simulink library "SimulationLibrary"  (R2016b)
settings: Solver=ode45  StartTime=0.0  StopTime=10.0  RelTol=1e-3  EnableMultiTasking=on
values from neighbouring files (symbols this model uses):
  cassieEtherCatData = cassieEtherCat.getStructure    [simulationInitFcn.m]
  pelvisPosition = [0; 0; 1.01]    [simulationInitFcn.m]
undefined symbols (not defined in the file or in its folder): CassieParameters, leftFootDrive, leftLegMedulla, pelvisMedulla, X, Y, Z
libraries: sm_lib x86, SimulationLibrary x30, nesl_utility x18, Contact_Forces_Lib x2
(part 3 of 3)

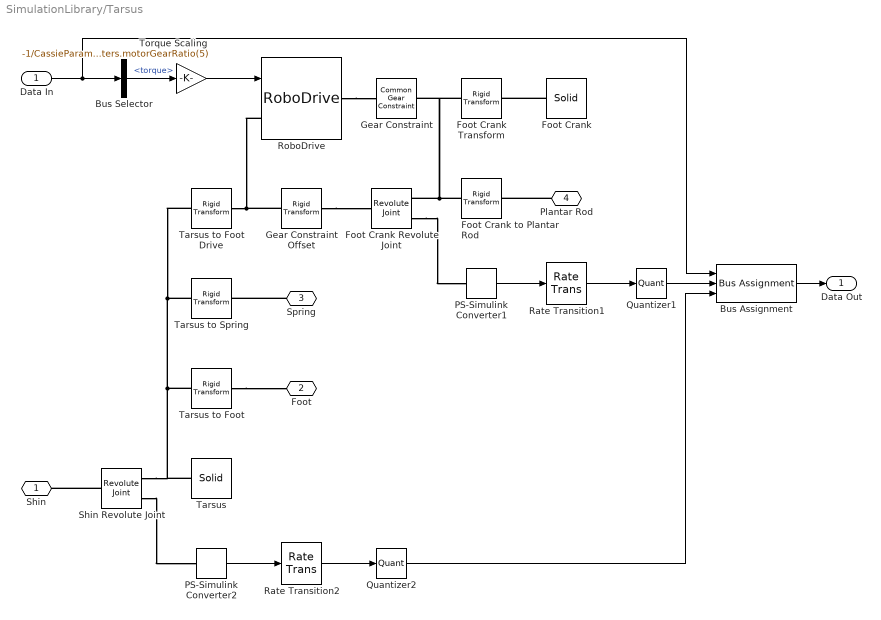
== system SimulationLibrary/Tarsus ==
  Data In : Inport  OutDataTypeStr=Bus: cassieEtherCatBus
  Bus Assignment : BusAssignment  AssignedSignals=leftFootDrive.inputs.position,leftLegMedulla.miscInputs.ankleJointEncoder
  Bus Selector : BusSelector  OutputSignals=leftFootDrive.outputs.torque
  Foot Crank : sm_lib/Body Elements/Solid  InertiaType=Custom  Mass=0.129  MassUnits=kg  CenterOfMass=[4.81; 0.02; -2.93]/1000  CenterOfMassUnits=m  MomentsOfInertia=[30.7; 57.05; 66.43]/1000000  MomentsOfInertiaUnits=kg*m^2  ProductsOfInertia=[0.0066; 2.62; 0.0019]/1000000  ProductsOfInertiaUnits=kg*m^2  DensityBased=on  Density=1000  DensityUnits=kg/(m^3)  DoExposeReferenceFrame=on  SerializedFrames=<Frames/>  GraphicType=FromGeometry  MarkerShape=Sphere  MarkerSize=10  GraphicVisPropType=AdvancedVisualProperties  GraphicDiffuseColor=simulationParameters.diffuseColor  GraphicSpecularColor=simulationParameters.specularColor  GraphicAmbientColor=simulationParameters.ambientColor  GraphicEmissiveColor=simulationParameters.emissiveColor  GraphicShininess=simulationParameters.shininess  GraphicOpacity=1  GeometryShape=FromFile  RectangleSize=[1 1]  RectangleSizeUnits=m  BrickDimensions=[1 1 1]  BrickDimensionUnits=m  CylinderRadius=1  CylinderRadiusUnits=m  CylinderLength=1  CylinderLengthUnits=m  SphereRadius=1  SphereRadiusUnits=m  EllipsoidRadii=[1 1 1]  EllipsoidRadiiUnits=m  ExtrusionCrossSection=[1 1; -1 1; -1 -1; 1 -1]  ExtrusionCrossSectionUnits=m  ExtrusionLength=1  ExtrusionLengthUnits=m  PolygonNumSides=3  PolygonOuterRadius=1  PolygonOuterRadiusUnits=m  ExtGeomFileType=STL  ExtGeomFileName=foot_crank.stl  ExtGeomFileUnits=m  RevolutionCrossSection=[1 1; 1 -1; 2 -1; 2 1]  RevolutionCrossSectionUnits=m  RevolutionExtent=Full  RevolutionAngle=180  RevolutionAngleUnits=deg
  Foot Crank Revolute Joint : sm_lib/Joints/Revolute Joint  SenseConstraintForce=off  SenseConstraintForceX=off  SenseConstraintForceY=off  SenseConstraintForceZ=off  SenseConstraintTorque=off  SenseConstraintTorqueX=off  SenseConstraintTorqueY=off  SenseConstraintTorqueZ=off  SenseTotalForce=off  SenseTotalForceX=off  SenseTotalForceY=off  SenseTotalForceZ=off  SenseTotalTorque=off  SenseTotalTorqueX=off  SenseTotalTorqueY=off  SenseTotalTorqueZ=off  CompositeWrenchDir=FollowerOnBase  CompositeWrenchFrame=BaseFrame  EquilibriumPosition=0  EquilibriumPositionUnits=deg  SpringStiffness=0  SpringStiffnessUnits=N*m/deg  DampingCoefficient=CassieParameters.motorViscousFrictionCoefficient(5)  DampingCoefficientUnits=N*m/(rad/s)  TorqueActuationMode=NoTorque  MotionActuationMode=ComputedMotion  SensePosition=on  SenseVelocity=off  SenseAcceleration=off  SenseTorqueForce=off  PositionTargetSpecify=on  PositionTargetPriority=High  PositionTargetValue=cassieEtherCatData.leftFootDrive.inputs.position  PositionTargetValueUnits=rad  VelocityTargetSpecify=on  VelocityTargetPriority=High  VelocityTargetValue=0  VelocityTargetValueUnits=rad/s
  Foot Crank Transform : sm_lib/Frames and Transforms/Rigid Transform  TranslationMethod=None  TranslationStandardOffset=0  TranslationLengthUnit=m  TranslationStandardAxis=+Z  TranslationCartesianOffset=[0 0 0]  TranslationROffset=0  TranslationROffsetUnits=m  TranslationZOffset=0  TranslationZOffsetUnits=m  TranslationThetaOffset=0  TranslationThetaOffsetUnits=deg  RotationMethod=StandardAxis  RotationAngleUnits=rad  RotationStandardAxis=+X  RotationAngle=0  RotationArbitraryAxis=[0 0 1]  FollAlignAxisA=+X  BaseAlignAxisA=+Y  FollAlignAxisB=+Y  BaseAlignAxisB=+Z  RotationSequenceAxes=FollowerAxes  RotationSequence=XYZ  RotationSequenceAngles=[90 0 0]  RotationSequenceAnglesUnits=deg  RotationMatrix=[1 0 0; 0 1 0; 0 0 1]
  Foot Crank to Plantar Rod : sm_lib/Frames and Transforms/Rigid Transform  TranslationMethod=Cartesian  TranslationStandardOffset=0  TranslationLengthUnit=m  TranslationStandardAxis=+Z  TranslationCartesianOffset=[55 0 -7.91]/1000  TranslationROffset=0  TranslationROffsetUnits=m  TranslationZOffset=0  TranslationZOffsetUnits=m  TranslationThetaOffset=0  TranslationThetaOffsetUnits=deg  RotationMethod=None  RotationAngleUnits=deg  RotationStandardAxis=+Z  RotationAngle=0.0  RotationArbitraryAxis=[0 0 1]  FollAlignAxisA=+X  BaseAlignAxisA=+Y  FollAlignAxisB=+Y  BaseAlignAxisB=+Z  RotationSequenceAxes=FollowerAxes  RotationSequence=XYZ  RotationSequenceAngles=[90 0 0]  RotationSequenceAnglesUnits=deg  RotationMatrix=[1 0 0; 0 1 0; 0 0 1]
  Gear Constraint : sm_lib/Gears and Couplings/Gears/Common Gear Constraint  GearType=External  SpecificationType=CenterDistanceRatio  CenterDistance=1e-6  CenterDistanceUnits=m  GearRatio=CassieParameters.motorGearRatio(5)  BaseGearRadius=10.0  BaseGearRadiusUnits=cm  FollGearRadius=10.0  FollGearRadiusUnits=cm  AssemblyGearRotation=Free
  Gear Constraint Offset : sm_lib/Frames and Transforms/Rigid Transform  TranslationMethod=StandardAxis  TranslationStandardOffset=1e-6  TranslationLengthUnit=m  TranslationStandardAxis=+Y  TranslationCartesianOffset=[0 0 0]  TranslationROffset=0  TranslationROffsetUnits=m  TranslationZOffset=0  TranslationZOffsetUnits=m  TranslationThetaOffset=0  TranslationThetaOffsetUnits=deg  RotationMethod=None  RotationAngleUnits=deg  RotationStandardAxis=+Z  RotationAngle=0.0  RotationArbitraryAxis=[0 0 1]  FollAlignAxisA=+X  BaseAlignAxisA=+Y  FollAlignAxisB=+Y  BaseAlignAxisB=+Z  RotationSequenceAxes=FollowerAxes  RotationSequence=XYX  RotationSequenceAngles=[0 0 0]  RotationSequenceAnglesUnits=deg  RotationMatrix=[1 0 0; 0 1 0; 0 0 1]
  PS-Simulink Converter1 : nesl_utility/PS-Simulink Converter  PhysicalDomain=network_engine_domain  SubClassName=ps_output  LeftPortType=input  RightPortType=output  PseudoPeriodic=off  Frequencies=[]  Unit=rad  AffineConversion=off
  PS-Simulink Converter2 : nesl_utility/PS-Simulink Converter  PhysicalDomain=network_engine_domain  SubClassName=ps_output  LeftPortType=input  RightPortType=output  PseudoPeriodic=off  Frequencies=[]  Unit=rad  AffineConversion=off
  Quantizer1 : Quantizer  QuantizationInterval=(2*pi)/(CassieParameters.motorEncoderTicks(5)*CassieParameters.motorGearRatio(5))
  Quantizer2 : Quantizer  QuantizationInterval=(2*pi)/CassieParameters.jointEncoderTicks(2)
  Rate Transition1 : RateTransition  Deterministic=off  OutPortSampleTime=CassieParameters.etherCatSampleTime
  Rate Transition2 : RateTransition  Deterministic=off  OutPortSampleTime=CassieParameters.etherCatSampleTime
  RoboDrive : SimulationLibrary/RoboDrive  model=50x8
  Shin Revolute Joint : sm_lib/Joints/Revolute Joint  SenseConstraintForce=off  SenseConstraintForceX=off  SenseConstraintForceY=off  SenseConstraintForceZ=off  SenseConstraintTorque=off  SenseConstraintTorqueX=off  SenseConstraintTorqueY=off  SenseConstraintTorqueZ=off  SenseTotalForce=off  SenseTotalForceX=off  SenseTotalForceY=off  SenseTotalForceZ=off  SenseTotalTorque=off  SenseTotalTorqueX=off  SenseTotalTorqueY=off  SenseTotalTorqueZ=off  CompositeWrenchDir=FollowerOnBase  CompositeWrenchFrame=BaseFrame  EquilibriumPosition=0  EquilibriumPositionUnits=deg  SpringStiffness=0  SpringStiffnessUnits=N*m/deg  DampingCoefficient=0  DampingCoefficientUnits=N*m/(deg/s)  TorqueActuationMode=NoTorque  MotionActuationMode=ComputedMotion  SensePosition=on  SenseVelocity=off  SenseAcceleration=off  SenseTorqueForce=off  PositionTargetSpecify=on  PositionTargetPriority=Low  PositionTargetValue=pi/2  PositionTargetValueUnits=rad  VelocityTargetSpecify=on  VelocityTargetPriority=High  VelocityTargetValue=0  VelocityTargetValueUnits=rad/s
  Tarsus : sm_lib/Body Elements/Solid  InertiaType=Custom  Mass=0.782  MassUnits=kg  CenterOfMass=[110.46; -30.58; -1.31]/1000  CenterOfMassUnits=m  MomentsOfInertia=[1125; 23138; 23947]/1000000  MomentsOfInertiaUnits=kg*m^2  ProductsOfInertia=[36.15; -63.29; -2878]/1000000  ProductsOfInertiaUnits=kg*m^2  DensityBased=on  Density=1000  DensityUnits=kg/(m^3)  DoExposeReferenceFrame=on  SerializedFrames=<Frames/>  GraphicType=FromGeometry  MarkerShape=Sphere  MarkerSize=10  GraphicVisPropType=AdvancedVisualProperties  GraphicDiffuseColor=simulationParameters.diffuseColor  GraphicSpecularColor=simulationParameters.specularColor  GraphicAmbientColor=simulationParameters.ambientColor  GraphicEmissiveColor=simulationParameters.emissiveColor  GraphicShininess=simulationParameters.shininess  GraphicOpacity=1.0  GeometryShape=FromFile  RectangleSize=[1 1]  RectangleSizeUnits=m  BrickDimensions=[1 1 1]  BrickDimensionUnits=m  CylinderRadius=1  CylinderRadiusUnits=m  CylinderLength=1  CylinderLengthUnits=m  SphereRadius=1  SphereRadiusUnits=m  EllipsoidRadii=[1 1 1]  EllipsoidRadiiUnits=m  ExtrusionCrossSection=[1 1; -1 1; -1 -1; 1 -1]  ExtrusionCrossSectionUnits=m  ExtrusionLength=1  ExtrusionLengthUnits=m  PolygonNumSides=3  PolygonOuterRadius=1  PolygonOuterRadiusUnits=m  ExtGeomFileType=STL  ExtGeomFileName=left_tarsus.stl  ExtGeomFileUnits=m  RevolutionCrossSection=[1 1; 1 -1; 2 -1; 2 1]  RevolutionCrossSectionUnits=m  RevolutionExtent=Full  RevolutionAngle=180  RevolutionAngleUnits=deg
  Tarsus to Foot : sm_lib/Frames and Transforms/Rigid Transform  TranslationMethod=Cartesian  TranslationStandardOffset=0  TranslationLengthUnit=m  TranslationStandardAxis=+Z  TranslationCartesianOffset=[408 -40 0]/1000  TranslationROffset=0  TranslationROffsetUnits=m  TranslationZOffset=0  TranslationZOffsetUnits=m  TranslationThetaOffset=0  TranslationThetaOffsetUnits=deg  RotationMethod=None  RotationAngleUnits=deg  RotationStandardAxis=+Z  RotationAngle=0.0  RotationArbitraryAxis=[0 0 1]  FollAlignAxisA=+X  BaseAlignAxisA=+Y  FollAlignAxisB=+Y  BaseAlignAxisB=+Z  RotationSequenceAxes=FollowerAxes  RotationSequence=XYZ  RotationSequenceAngles=[-90 0 0]  RotationSequenceAnglesUnits=deg  RotationMatrix=[1 0 0; 0 1 0; 0 0 1]
  Tarsus to Foot Drive : sm_lib/Frames and Transforms/Rigid Transform  TranslationMethod=Cartesian  TranslationStandardOffset=0  TranslationLengthUnit=m  TranslationStandardAxis=+Z  TranslationCartesianOffset=[58 -34 22.75]/1000  TranslationROffset=0  TranslationROffsetUnits=m  TranslationZOffset=0  TranslationZOffsetUnits=m  TranslationThetaOffset=0  TranslationThetaOffsetUnits=deg  RotationMethod=None  RotationAngleUnits=deg  RotationStandardAxis=+Z  RotationAngle=0  RotationArbitraryAxis=[0 0 1]  FollAlignAxisA=+X  BaseAlignAxisA=+Y  FollAlignAxisB=+Y  BaseAlignAxisB=+Z  RotationSequenceAxes=FollowerAxes  RotationSequence=XYZ  RotationSequenceAngles=[-90 0 0]  RotationSequenceAnglesUnits=deg  RotationMatrix=[1 0 0; 0 1 0; 0 0 1]
  Tarsus to Spring : sm_lib/Frames and Transforms/Rigid Transform  TranslationMethod=Cartesian  TranslationStandardOffset=0  TranslationLengthUnit=m  TranslationStandardAxis=+Z  TranslationCartesianOffset=[-12.69 -30.59 0.92]/1000  TranslationROffset=0  TranslationROffsetUnits=m  TranslationZOffset=0  TranslationZOffsetUnits=m  TranslationThetaOffset=0  TranslationThetaOffsetUnits=deg  RotationMethod=RotationSequence  RotationAngleUnits=deg  RotationStandardAxis=+Z  RotationAngle=0.0  RotationArbitraryAxis=[0 0 1]  FollAlignAxisA=+X  BaseAlignAxisA=+Y  FollAlignAxisB=+Y  BaseAlignAxisB=+Z  RotationSequenceAxes=BaseAxes  RotationSequence=ZYX  RotationSequenceAngles=[155.8, 0.315, 4.47]  RotationSequenceAnglesUnits=deg  RotationMatrix=eye(3)
  Torque Scaling : Gain  Gain=-1/CassieParameters.motorGearRatio(5)
  Shin : PMIOPort  Port=1  Side=Left
  Foot : PMIOPort  Port=2  Side=Right
  Spring : PMIOPort  Port=3  Side=Left
  Plantar Rod : PMIOPort  Port=4  Side=Right
  Data Out : Outport
  wires:
  Bus Assignment/1 -> Data Out/1
  Data In/1 -> Bus Selector/1, Bus Assignment/1
  PS-Simulink Converter2/1 -> Rate Transition2/1
  PS-Simulink Converter1/1 -> Rate Transition1/1
  Bus Selector/1 -> Torque Scaling/1  "<torque>"
  Torque Scaling/1 -> RoboDrive/1
  Rate Transition1/1 -> Quantizer1/1
  Quantizer1/1 -> Bus Assignment/2
  Rate Transition2/1 -> Quantizer2/1
  Quantizer2/1 -> Bus Assignment/3
  connections:
  Tarsus to Foot/RConn1 -- Foot/RConn1
  Spring/RConn1 -- Tarsus to Spring/RConn1
  Shin Revolute Joint/LConn1 -- Shin/RConn1
  Shin Revolute Joint/RConn2 -- PS-Simulink Converter2/LConn1
  Tarsus to Foot/LConn1 -- Shin Revolute Joint/RConn1 -- Tarsus/RConn1 -- Tarsus to Foot Drive/LConn1 -- Tarsus to Spring/LConn1
  Tarsus to Foot Drive/RConn1 -- Gear Constraint Offset/LConn1 -- RoboDrive/LConn1
  RoboDrive/RConn1 -- Gear Constraint/LConn1
  Gear Constraint Offset/RConn1 -- Foot Crank Revolute Joint/LConn1
  Foot Crank to Plantar Rod/LConn1 -- Foot Crank Revolute Joint/RConn1 -- Foot Crank Transform/LConn1 -- Gear Constraint/RConn1
  Plantar Rod/RConn1 -- Foot Crank to Plantar Rod/RConn1
  Foot Crank Revolute Joint/RConn2 -- PS-Simulink Converter1/LConn1
  Foot Crank/RConn1 -- Foot Crank Transform/RConn1

== system SimulationLibrary/Thigh ==
  Data In : Inport
  Thigh : sm_lib/Body Elements/Solid  InertiaType=Custom  Mass=5.52  MassUnits=kg  CenterOfMass=[59.46; 0.05; -35.81]/1000  CenterOfMassUnits=m  MomentsOfInertia=[17969; 56284; 49756]/1000000  MomentsOfInertiaUnits=kg*m^2  ProductsOfInertia=[-19.26; -11685; 283.6]/1000000  ProductsOfInertiaUnits=kg*m^2  DensityBased=on  Density=1000  DensityUnits=kg/(m^3)  DoExposeReferenceFrame=on  SerializedFrames=<Frames/>  GraphicType=FromGeometry  MarkerShape=Sphere  MarkerSize=10  MarkerSizeUnits=m  GraphicVisPropType=AdvancedVisualProperties  GraphicDiffuseColor=simulationParameters.diffuseColor  GraphicSpecularColor=simulationParameters.specularColor  GraphicAmbientColor=simulationParameters.ambientColor  GraphicEmissiveColor=simulationParameters.emissiveColor  GraphicShininess=simulationParameters.shininess  GraphicOpacity=1  GeometryShape=FromFile  RectangleSize=[1 1]  RectangleSizeUnits=m  BrickDimensions=[0.15 0.15 0.2]  BrickDimensionUnits=m  CylinderRadius=0.05  CylinderRadiusUnits=m  CylinderLength=0.1  CylinderLengthUnits=m  SphereRadius=1  SphereRadiusUnits=m  EllipsoidRadii=[1 1 1]  EllipsoidRadiiUnits=m  ExtrusionCrossSection=[1 1; -1 1; -1 -1; 1 -1]  ExtrusionCrossSectionUnits=m  ExtrusionLength=1  ExtrusionLengthUnits=m  PolygonNumSides=3  PolygonOuterRadius=1  PolygonOuterRadiusUnits=m  ExtGeomFileType=STL  ExtGeomFileName=left_thigh.stl  ExtGeomFileUnits=m  RevolutionCrossSection=[1 1; 1 -1; 2 -1; 2 1]  RevolutionCrossSectionUnits=m  RevolutionExtent=Full  RevolutionAngle=180  RevolutionAngleUnits=deg
  Thigh to Achilles : sm_lib/Frames and Transforms/Rigid Transform  TranslationMethod=Cartesian  TranslationStandardOffset=0  TranslationLengthUnit=m  TranslationStandardAxis=+Z  TranslationCartesianOffset=[0, 0, 0.045]  TranslationROffset=0  TranslationROffsetUnits=m  TranslationZOffset=0  TranslationZOffsetUnits=m  TranslationThetaOffset=0  TranslationThetaOffsetUnits=deg  RotationMethod=None  RotationAngleUnits=deg  RotationStandardAxis=+Z  RotationAngle=0.0  RotationArbitraryAxis=[0 0 1]  FollAlignAxisA=+X  BaseAlignAxisA=+Y  FollAlignAxisB=+Y  BaseAlignAxisB=+Z  RotationSequenceAxes=FollowerAxes  RotationSequence=XYX  RotationSequenceAngles=[0 0 0]  RotationSequenceAnglesUnits=deg  RotationMatrix=[1 0 0; 0 1 0; 0 0 1]
  Thigh to Knee : sm_lib/Frames and Transforms/Rigid Transform  TranslationMethod=Cartesian  TranslationStandardOffset=0  TranslationLengthUnit=m  TranslationStandardAxis=+Z  TranslationCartesianOffset=[0.12, 0, 0.0045]  TranslationROffset=0  TranslationROffsetUnits=m  TranslationZOffset=0  TranslationZOffsetUnits=m  TranslationThetaOffset=0  TranslationThetaOffsetUnits=deg  RotationMethod=None  RotationAngleUnits=deg  RotationStandardAxis=+Z  RotationAngle=0.0  RotationArbitraryAxis=[0 0 1]  FollAlignAxisA=+X  BaseAlignAxisA=+Y  FollAlignAxisB=+Y  BaseAlignAxisB=+Z  RotationSequenceAxes=FollowerAxes  RotationSequence=XYX  RotationSequenceAngles=[0 0 0]  RotationSequenceAnglesUnits=deg  RotationMatrix=[1 0 0; 0 1 0; 0 0 1]
  Hip : PMIOPort  Port=1  Side=Left
  Knee : PMIOPort  Port=2  Side=Right
  Achilles : PMIOPort  Port=3  Side=Right
  Data Out : Outport
  wires:
  Data In/1 -> Data Out/1
  connections:
  Hip/RConn1 -- Thigh to Knee/LConn1 -- Thigh to Achilles/LConn1 -- Thigh/RConn1
  Thigh to Knee/RConn1 -- Knee/RConn1
  Achilles/RConn1 -- Thigh to Achilles/RConn1

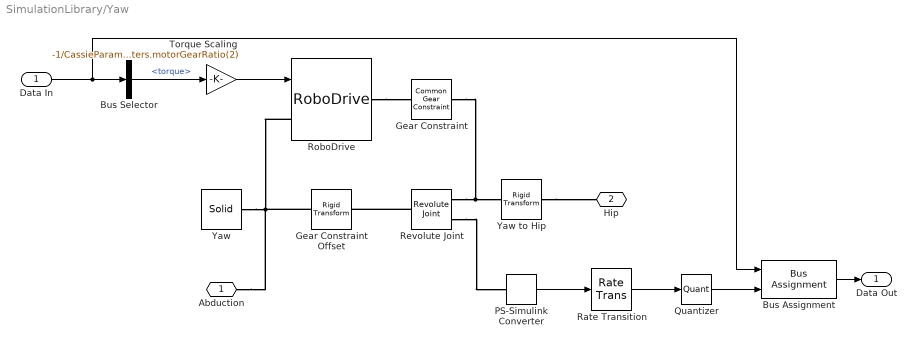
== system SimulationLibrary/Yaw ==
  Data In : Inport  OutDataTypeStr=Bus: cassieEtherCatBus
  Bus Assignment : BusAssignment  AssignedSignals=leftYawDrive.inputs.position
  Bus Selector : BusSelector  OutputSignals=leftYawDrive.outputs.torque
  Gear Constraint : sm_lib/Gears and Couplings/Gears/Common Gear Constraint  GearType=External  SpecificationType=CenterDistanceRatio  CenterDistance=1e-6  CenterDistanceUnits=m  GearRatio=CassieParameters.motorGearRatio(2)  BaseGearRadius=10.0  BaseGearRadiusUnits=cm  FollGearRadius=10.0  FollGearRadiusUnits=cm  AssemblyGearRotation=Free
  Gear Constraint Offset : sm_lib/Frames and Transforms/Rigid Transform  TranslationMethod=StandardAxis  TranslationStandardOffset=1e-6  TranslationLengthUnit=m  TranslationStandardAxis=+Y  TranslationCartesianOffset=[0 0 0]  TranslationROffset=0  TranslationROffsetUnits=m  TranslationZOffset=0  TranslationZOffsetUnits=m  TranslationThetaOffset=0  TranslationThetaOffsetUnits=deg  RotationMethod=None  RotationAngleUnits=deg  RotationStandardAxis=+Z  RotationAngle=0.0  RotationArbitraryAxis=[0 0 1]  FollAlignAxisA=+X  BaseAlignAxisA=+Y  FollAlignAxisB=+Y  BaseAlignAxisB=+Z  RotationSequenceAxes=FollowerAxes  RotationSequence=XYX  RotationSequenceAngles=[0 0 0]  RotationSequenceAnglesUnits=deg  RotationMatrix=[1 0 0; 0 1 0; 0 0 1]
  PS-Simulink Converter : nesl_utility/PS-Simulink Converter  PhysicalDomain=network_engine_domain  SubClassName=ps_output  LeftPortType=input  RightPortType=output  PseudoPeriodic=off  Frequencies=[]  Unit=rad  AffineConversion=off
  Quantizer : Quantizer  QuantizationInterval=(2*pi)/(CassieParameters.motorEncoderTicks(2)*CassieParameters.motorGearRatio(2))
  Rate Transition : RateTransition  Deterministic=off  OutPortSampleTime=CassieParameters.etherCatSampleTime
  Revolute Joint : sm_lib/Joints/Revolute Joint  SenseConstraintForce=off  SenseConstraintForceX=off  SenseConstraintForceY=off  SenseConstraintForceZ=off  SenseConstraintTorque=off  SenseConstraintTorqueX=off  SenseConstraintTorqueY=off  SenseConstraintTorqueZ=off  SenseTotalForce=off  SenseTotalForceX=off  SenseTotalForceY=off  SenseTotalForceZ=off  SenseTotalTorque=off  SenseTotalTorqueX=off  SenseTotalTorqueY=off  SenseTotalTorqueZ=off  CompositeWrenchDir=FollowerOnBase  CompositeWrenchFrame=BaseFrame  EquilibriumPosition=0  EquilibriumPositionUnits=rad  SpringStiffness=0  SpringStiffnessUnits=N*m/rad  DampingCoefficient=CassieParameters.motorViscousFrictionCoefficient(2)  DampingCoefficientUnits=N*m/(rad/s)  TorqueActuationMode=NoTorque  MotionActuationMode=ComputedMotion  SensePosition=on  SenseVelocity=off  SenseAcceleration=off  SenseTorqueForce=off  PositionTargetSpecify=on  PositionTargetPriority=High  PositionTargetValue=cassieEtherCatData.leftYawDrive.inputs.position  PositionTargetValueUnits=rad  VelocityTargetSpecify=on  VelocityTargetPriority=High  VelocityTargetValue=0  VelocityTargetValueUnits=rad/s
  RoboDrive : SimulationLibrary/RoboDrive  model=85x13
  Torque Scaling : Gain  Gain=-1/CassieParameters.motorGearRatio(2)
  Yaw : sm_lib/Body Elements/Solid  InertiaType=Custom  Mass=1.82  MassUnits=kg  CenterOfMass=[25.7; 0.1; 17.93]/1000  CenterOfMassUnits=m  MomentsOfInertia=[2722; 5586; 4638]/1000000  MomentsOfInertiaUnits=kg*m^2  ProductsOfInertia=[2.61; 1.53; 0.703]/1000000  ProductsOfInertiaUnits=kg*m^2  DensityBased=on  Density=1000  DensityUnits=kg/(m^3)  DoExposeReferenceFrame=on  SerializedFrames=<Frames/>  GraphicType=FromGeometry  MarkerShape=Sphere  MarkerSize=10  MarkerSizeUnits=m  GraphicVisPropType=AdvancedVisualProperties  GraphicDiffuseColor=simulationParameters.diffuseColor  GraphicSpecularColor=simulationParameters.specularColor  GraphicAmbientColor=simulationParameters.ambientColor  GraphicEmissiveColor=simulationParameters.emissiveColor  GraphicShininess=simulationParameters.shininess  GraphicOpacity=1  GeometryShape=FromFile  RectangleSize=[1 1]  RectangleSizeUnits=m  BrickDimensions=[0.15 0.15 0.2]  BrickDimensionUnits=m  CylinderRadius=0.05  CylinderRadiusUnits=m  CylinderLength=0.1  CylinderLengthUnits=m  SphereRadius=1  SphereRadiusUnits=m  EllipsoidRadii=[1 1 1]  EllipsoidRadiiUnits=m  ExtrusionCrossSection=[1 1; -1 1; -1 -1; 1 -1]  ExtrusionCrossSectionUnits=m  ExtrusionLength=1  ExtrusionLengthUnits=m  PolygonNumSides=3  PolygonOuterRadius=1  PolygonOuterRadiusUnits=m  ExtGeomFileType=STL  ExtGeomFileName=left_yaw.stl  ExtGeomFileUnits=m  RevolutionCrossSection=[1 1; 1 -1; 2 -1; 2 1]  RevolutionCrossSectionUnits=m  RevolutionExtent=Full  RevolutionAngle=180  RevolutionAngleUnits=deg
  Yaw to Hip : sm_lib/Frames and Transforms/Rigid Transform  TranslationMethod=Cartesian  TranslationStandardOffset=0  TranslationLengthUnit=m  TranslationStandardAxis=+Z  TranslationCartesianOffset=[0, 0, -0.09]  TranslationROffset=0  TranslationROffsetUnits=m  TranslationZOffset=0  TranslationZOffsetUnits=m  TranslationThetaOffset=0  TranslationThetaOffsetUnits=deg  RotationMethod=RotationMatrix  RotationAngleUnits=deg  RotationStandardAxis=+Z  RotationAngle=0.0  RotationArbitraryAxis=[0 0 1]  FollAlignAxisA=+X  BaseAlignAxisA=+Y  FollAlignAxisB=+Y  BaseAlignAxisB=+Z  RotationSequenceAxes=FollowerAxes  RotationSequence=XYZ  RotationSequenceAngles=[90 0 0]  RotationSequenceAnglesUnits=deg  RotationMatrix=[0, 1, 0; 0, 0, -1; -1, 0, 0]
  Abduction : PMIOPort  Port=1  Side=Left
  Hip : PMIOPort  Port=2  Side=Right
  Data Out : Outport
  wires:
  Torque Scaling/1 -> RoboDrive/1
  Data In/1 -> Bus Selector/1, Bus Assignment/1
  Bus Assignment/1 -> Data Out/1
  Rate Transition/1 -> Quantizer/1
  Bus Selector/1 -> Torque Scaling/1  "<torque>"
  PS-Simulink Converter/1 -> Rate Transition/1
  Quantizer/1 -> Bus Assignment/2
  connections:
  Yaw/RConn1 -- RoboDrive/LConn1 -- Abduction/RConn1 -- Gear Constraint Offset/LConn1
  Revolute Joint/LConn1 -- Gear Constraint Offset/RConn1
  RoboDrive/RConn1 -- Gear Constraint/LConn1
  Gear Constraint/RConn1 -- Revolute Joint/RConn1 -- Yaw to Hip/LConn1
  Revolute Joint/RConn2 -- PS-Simulink Converter/LConn1
  Yaw to Hip/RConn1 -- Hip/RConn1

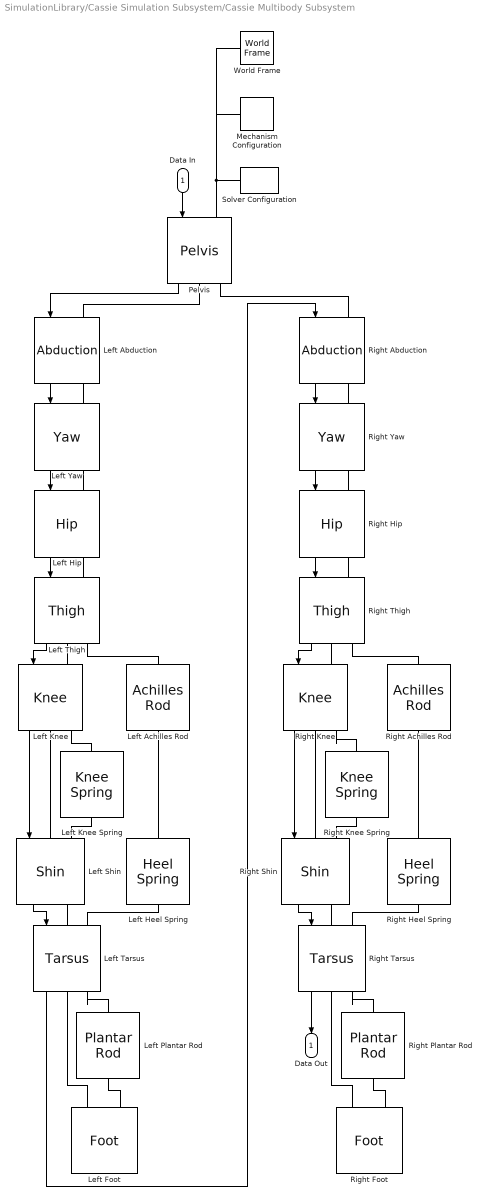
== system SimulationLibrary/Cassie Simulation Subsystem/Cassie Multibody Subsystem ==
  Data In : Inport  PortDimensions=1
  Left Abduction : SimulationLibrary/Abduction  side=Left
  Left Achilles Rod : SimulationLibrary/Achilles Rod  SystemSampleTime=-1
  Left Foot : SimulationLibrary/Foot  side=Left
  Left Heel Spring : SimulationLibrary/Heel Spring
  Left Hip : SimulationLibrary/Hip  side=Left
  Left Knee : SimulationLibrary/Knee  side=Left
  Left Knee Spring : SimulationLibrary/Knee Spring
  Left Plantar Rod : SimulationLibrary/Plantar Rod  SystemSampleTime=-1
  Left Shin : SimulationLibrary/Shin  side=Left
  Left Tarsus : SimulationLibrary/Tarsus  side=Left
  Left Thigh : SimulationLibrary/Thigh  side=Left
  Left Yaw : SimulationLibrary/Yaw  side=Left
  Mechanism Configuration : sm_lib/Utilities/Mechanism Configuration  UniformGravity=Constant  GravityVector=simulationParameters.gravity  GravityUnits=m/s^2  LinearizationDelta=0.001
  Pelvis : SimulationLibrary/Pelvis  SystemSampleTime=-1
  Right Abduction : SimulationLibrary/Abduction  side=Right
  Right Achilles Rod : SimulationLibrary/Achilles Rod  SystemSampleTime=-1
  Right Foot : SimulationLibrary/Foot  side=Right
  Right Heel Spring : SimulationLibrary/Heel Spring
  Right Hip : SimulationLibrary/Hip  side=Right
  Right Knee : SimulationLibrary/Knee  side=Right
  Right Knee Spring : SimulationLibrary/Knee Spring
  Right Plantar Rod : SimulationLibrary/Plantar Rod  SystemSampleTime=-1
  Right Shin : SimulationLibrary/Shin  side=Right
  Right Tarsus : SimulationLibrary/Tarsus  side=Right
  Right Thigh : SimulationLibrary/Thigh  side=Right
  Right Yaw : SimulationLibrary/Yaw  side=Right
  Solver Configuration : nesl_utility/Solver Configuration  PhysicalDomain=network_engine_domain  SubClassName=solver  LeftPortType=input  RightPortType=generic  Accelerate=off  Tones=[]  Harmonics=[]  SimulateNoise=off  Profile=off  UseLocalSampling=off  EnableSwitchedLinearOptims=on  FrequencyDomain=off  UseCCode=off  RelTol=0.001  AbsTol=1e-06  MinStep=1e-09  ToWorkspace=off  RevertToSquareIcSolve=off  NumHomotopyIterations=100  PhasorMode=off  PhasorModeNumHarmonics=1  OverrideAbsTol=off  DoDC=off  ResidualTolerance=1e-09  UseLocalSolver=off  LocalSolverChoice=NE_BACKWARD_EULER_ADVANCER  LocalSolverSampleTime=0.001  DoFixedCost=off  MaxNonlinIter=3  MaxModeIter=2  LinearAlgebra=Sparse  DelaysMemoryBudget=1024  AutomaticFiltering=on  FilteringTimeConstant=0.001
  World Frame : sm_lib/Frames and Transforms/World Frame
  Data Out : Outport  PortDimensions=1
  wires:
  Right Abduction/1 -> Right Yaw/1
  Left Abduction/1 -> Left Yaw/1
  Left Yaw/1 -> Left Hip/1
  Left Hip/1 -> Left Thigh/1
  Right Yaw/1 -> Right Hip/1
  Right Hip/1 -> Right Thigh/1
  Left Thigh/1 -> Left Knee/1
  Right Thigh/1 -> Right Knee/1
  Left Knee/1 -> Left Shin/1
  Data In/1 -> Pelvis/1
  Pelvis/1 -> Left Abduction/1
  Right Knee/1 -> Right Shin/1
  Left Shin/1 -> Left Tarsus/1
  Left Tarsus/1 -> Right Abduction/1
  Right Shin/1 -> Right Tarsus/1
  Right Tarsus/1 -> Data Out/1
  connections:
  Solver Configuration/RConn1 -- Pelvis/LConn1 -- Mechanism Configuration/RConn1 -- World Frame/RConn1
  Left Yaw/LConn1 -- Left Abduction/RConn1
  Right Yaw/LConn1 -- Right Abduction/RConn1
  Left Hip/LConn1 -- Left Yaw/RConn1
  Left Thigh/LConn1 -- Left Hip/RConn1
  Right Hip/LConn1 -- Right Yaw/RConn1
  Right Thigh/LConn1 -- Right Hip/RConn1
  Left Knee/LConn1 -- Left Thigh/RConn1
  Left Thigh/RConn2 -- Left Achilles Rod/LConn1
  Right Knee/LConn1 -- Right Thigh/RConn1
  Right Thigh/RConn2 -- Right Achilles Rod/LConn1
  Left Knee/RConn2 -- Left Knee Spring/LConn1
  Left Shin/LConn2 -- Left Knee Spring/RConn1
  Left Shin/LConn1 -- Left Knee/RConn1
  Left Achilles Rod/RConn1 -- Left Heel Spring/RConn1
  Right Knee/RConn2 -- Right Knee Spring/LConn1
  Right Shin/LConn2 -- Right Knee Spring/RConn1
  Right Shin/LConn1 -- Right Knee/RConn1
  Right Heel Spring/RConn1 -- Right Achilles Rod/RConn1
  Left Tarsus/LConn1 -- Left Shin/RConn1
  Left Tarsus/LConn2 -- Left Heel Spring/LConn1
  Left Tarsus/RConn2 -- Left Plantar Rod/LConn1
  Left Tarsus/RConn1 -- Left Foot/LConn1
  Right Abduction/LConn1 -- Pelvis/RConn2
  Left Abduction/LConn1 -- Pelvis/RConn1
  Right Tarsus/RConn2 -- Right Plantar Rod/LConn1
  Right Tarsus/RConn1 -- Right Foot/LConn1
  Right Tarsus/LConn1 -- Right Shin/RConn1
  Right Tarsus/LConn2 -- Right Heel Spring/LConn1
  Left Foot/LConn2 -- Left Plantar Rod/RConn1
  Right Foot/LConn2 -- Right Plantar Rod/RConn1

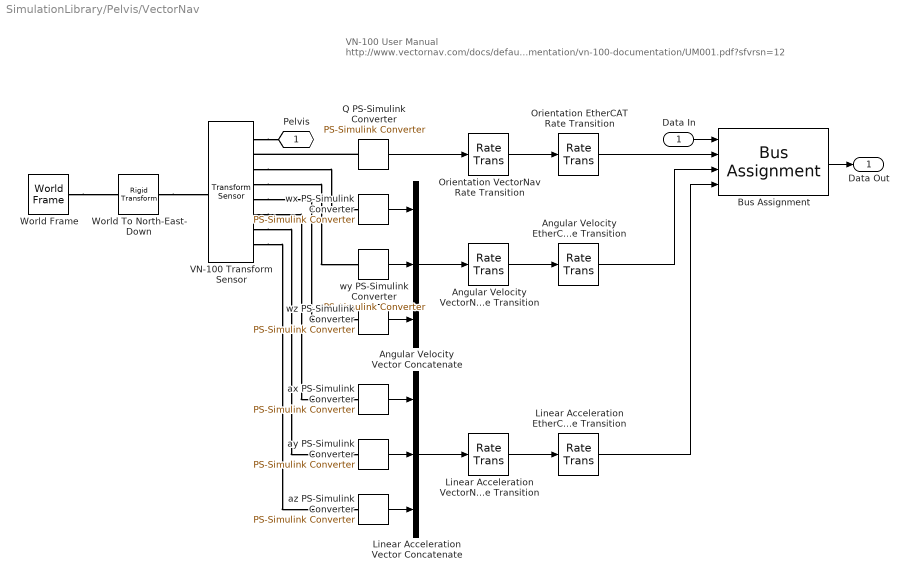
== system SimulationLibrary/Pelvis/VectorNav ==
  note: VN-100 User Manual
      | http://www.vectornav.com/docs/default-source/documentation/vn-100-documentation/UM001.pdf?sfvrsn=12
  Data In : Inport  OutDataTypeStr=Bus: cassieEtherCatBus
  Angular Velocity EtherCAT Rate Transition : RateTransition  Deterministic=off  OutPortSampleTime=CassieParameters.etherCatSampleTime
  Angular Velocity Vector Concatenate : Concatenate  NumInputs=3
  Angular Velocity VectorNav Rate Transition : RateTransition  Deterministic=off  OutPortSampleTime=CassieParameters.vectorNavSampleTime
  Bus Assignment : BusAssignment  AssignedSignals=pelvisMedulla.vnInputs.orientation,pelvisMedulla.vnInputs.angularVelocity,pelvisMedulla.vnInputs.linearAcceleration
  Linear Acceleration EtherCAT Rate Transition : RateTransition  Deterministic=off  OutPortSampleTime=CassieParameters.etherCatSampleTime
  Linear Acceleration Vector Concatenate : Concatenate  NumInputs=3
  Linear Acceleration VectorNav Rate Transition : RateTransition  Deterministic=off  OutPortSampleTime=CassieParameters.vectorNavSampleTime
  Orientation EtherCAT Rate Transition : RateTransition  Deterministic=off  OutPortSampleTime=CassieParameters.etherCatSampleTime
  Orientation VectorNav Rate Transition : RateTransition  Deterministic=off  OutPortSampleTime=CassieParameters.vectorNavSampleTime
  Q PS-Simulink Converter : nesl_utility/PS-Simulink Converter  PhysicalDomain=network_engine_domain  SubClassName=ps_output  LeftPortType=input  RightPortType=output  PseudoPeriodic=off  Frequencies=[]  Unit=1  AffineConversion=off
  VN-100 Transform Sensor : sm_lib/Frames and Transforms/Transform Sensor  MeasurementFrame=Follower  SenseAngle=off  SenseAxis=off  SenseAngle1=off  SenseAngle2=off  SenseAngle3=off  SenseQ=on  SenseR=off  SenseOmegaX=on  SenseOmegaY=on  SenseOmegaZ=on  SenseOmega1=off  SenseOmega2=off  SenseOmega3=off  SenseQDot=off  SenseRDot=off  SenseAlphaX=off  SenseAlphaY=off  SenseAlphaZ=off  SenseAlpha1=off  SenseAlpha2=off  SenseAlpha3=off  SenseQDDot=off  SenseRDDot=off  SenseX=off  SenseY=off  SenseZ=off  SenseRad=off  SenseAzim=off  SenseDist=off  SenseInc=off  SenseXDot=off  SenseYDot=off  SenseZDot=off  SenseRadDot=off  SenseAzimDot=off  SenseDistDot=off  SenseIncDot=off  SenseXDDot=on  SenseYDDot=on  SenseZDDot=on  SenseRadDDot=off  SenseAzimDDot=off  SenseDistDDot=off  SenseIncDDot=off
  World Frame : sm_lib/Frames and Transforms/World Frame
  World To North-East-Down : sm_lib/Frames and Transforms/Rigid Transform  TranslationMethod=None  TranslationStandardOffset=0  TranslationLengthUnit=m  TranslationStandardAxis=+Z  TranslationCartesianOffset=[0 0 0]  TranslationROffset=0  TranslationROffsetUnits=m  TranslationZOffset=0  TranslationZOffsetUnits=m  TranslationThetaOffset=0  TranslationThetaOffsetUnits=deg  RotationMethod=StandardAxis  RotationAngleUnits=deg  RotationStandardAxis=+X  RotationAngle=180  RotationArbitraryAxis=[0 0 1]  FollAlignAxisA=+X  BaseAlignAxisA=+Y  FollAlignAxisB=+Y  BaseAlignAxisB=+Z  RotationSequenceAxes=FollowerAxes  RotationSequence=XYX  RotationSequenceAngles=[0 0 0]  RotationSequenceAnglesUnits=deg  RotationMatrix=[1 0 0; 0 1 0; 0 0 1]
  ax PS-Simulink Converter : nesl_utility/PS-Simulink Converter  PhysicalDomain=network_engine_domain  SubClassName=ps_output  LeftPortType=input  RightPortType=output  PseudoPeriodic=off  Frequencies=[]  Unit=1  AffineConversion=off
  ay PS-Simulink Converter : nesl_utility/PS-Simulink Converter  PhysicalDomain=network_engine_domain  SubClassName=ps_output  LeftPortType=input  RightPortType=output  PseudoPeriodic=off  Frequencies=[]  Unit=1  AffineConversion=off
  az PS-Simulink Converter : nesl_utility/PS-Simulink Converter  PhysicalDomain=network_engine_domain  SubClassName=ps_output  LeftPortType=input  RightPortType=output  PseudoPeriodic=off  Frequencies=[]  Unit=1  AffineConversion=off
  wx PS-Simulink Converter : nesl_utility/PS-Simulink Converter  PhysicalDomain=network_engine_domain  SubClassName=ps_output  LeftPortType=input  RightPortType=output  PseudoPeriodic=off  Frequencies=[]  Unit=1  AffineConversion=off
  wy PS-Simulink Converter : nesl_utility/PS-Simulink Converter  PhysicalDomain=network_engine_domain  SubClassName=ps_output  LeftPortType=input  RightPortType=output  PseudoPeriodic=off  Frequencies=[]  Unit=1  AffineConversion=off
  wz PS-Simulink Converter : nesl_utility/PS-Simulink Converter  PhysicalDomain=network_engine_domain  SubClassName=ps_output  LeftPortType=input  RightPortType=output  PseudoPeriodic=off  Frequencies=[]  Unit=1  AffineConversion=off
  Pelvis : PMIOPort  Port=1  Side=Left
  Data Out : Outport
  wires:
  Linear Acceleration EtherCAT Rate Transition/1 -> Bus Assignment/4
  Angular Velocity EtherCAT Rate Transition/1 -> Bus Assignment/3
  Orientation EtherCAT Rate Transition/1 -> Bus Assignment/2
  Data In/1 -> Bus Assignment/1
  Bus Assignment/1 -> Data Out/1
  Q PS-Simulink Converter/1 -> Orientation VectorNav Rate Transition/1
  Orientation VectorNav Rate Transition/1 -> Orientation EtherCAT Rate Transition/1
  ay PS-Simulink Converter/1 -> Linear Acceleration Vector Concatenate/2
  ax PS-Simulink Converter/1 -> Linear Acceleration Vector Concatenate/1
  az PS-Simulink Converter/1 -> Linear Acceleration Vector Concatenate/3
  Linear Acceleration Vector Concatenate/1 -> Linear Acceleration VectorNav Rate Transition/1
  Linear Acceleration VectorNav Rate Transition/1 -> Linear Acceleration EtherCAT Rate Transition/1
  wy PS-Simulink Converter/1 -> Angular Velocity Vector Concatenate/2
  wx PS-Simulink Converter/1 -> Angular Velocity Vector Concatenate/1
  wz PS-Simulink Converter/1 -> Angular Velocity Vector Concatenate/3
  Angular Velocity Vector Concatenate/1 -> Angular Velocity VectorNav Rate Transition/1
  Angular Velocity VectorNav Rate Transition/1 -> Angular Velocity EtherCAT Rate Transition/1
  connections:
  Q PS-Simulink Converter/LConn1 -- VN-100 Transform Sensor/RConn2
  World To North-East-Down/RConn1 -- VN-100 Transform Sensor/LConn1
  VN-100 Transform Sensor/RConn1 -- Pelvis/RConn1
  World Frame/RConn1 -- World To North-East-Down/LConn1
  VN-100 Transform Sensor/RConn3 -- wx PS-Simulink Converter/LConn1
  VN-100 Transform Sensor/RConn4 -- wy PS-Simulink Converter/LConn1
  VN-100 Transform Sensor/RConn5 -- wz PS-Simulink Converter/LConn1
  VN-100 Transform Sensor/RConn6 -- ax PS-Simulink Converter/LConn1
  VN-100 Transform Sensor/RConn7 -- ay PS-Simulink Converter/LConn1
  VN-100 Transform Sensor/RConn8 -- az PS-Simulink Converter/LConn1

== matlab function SimulationLibrary/RoboDrive/Torque Speed Curve MATLAB Function ==
  data: speed input; torque input; torque output; peakTorque input; peakSpeed input
function torque = fcn(speed, torque, peakTorque, peakSpeed) %#codegen

  % Cap the velocity at the specified limits to avoid extrapolation
  speed = median([-peakSpeed, speed, peakSpeed]);

  % Linear interpolation of speed-torque curve
  torqueLimit = interp1(...
    [0, 0.5*peakSpeed, peakSpeed], ...
    [peakTorque, peakTorque, 0], ...
    abs(speed));

  % Cap the torque command at the specified imits
  torque = median([-torqueLimit, torque, torqueLimit]);
end % fcn
